simulink model "HysteresisFieldOrientedControl"  (R2020a)
settings: Solver=VariableStepAuto  StartTime=0.0  StopTime=10.0  RelTol=1e-3
libraries: simulink x1, powerlib_meascontrol x1
settings Model: Creator=Sony  LastModifiedBy=Sony

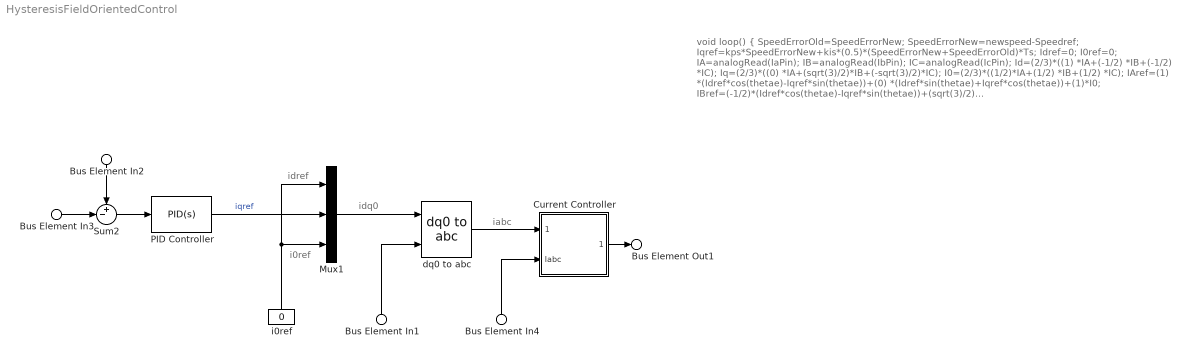
== system HysteresisFieldOrientedControl ==
  note: iabc
  note: idq0
  note: void loop()
      | {
      |   SpeedErrorOld=SpeedErrorNew;
      |   SpeedErrorNew=newspeed-Speedref;
      |
      |   Iqref=kps*SpeedErrorNew+kis*(0.5)*(SpeedErrorNew+SpeedErrorOld)*Ts;
      |   Idref=0;
      |   I0ref=0;
      |
      |   IA=analogRead(IaPin);
      |   IB=analogRead(IbPin);
      |   IC=analogRead(IcPin);
      |
      |   Id=(2/3)*((1)  *IA+(-1/2)     *IB+(-1/2)      *IC);
      |   Iq=(2/3)*((0)  *IA+(sqrt(3)/2)*IB+(-sqrt(3)/2)*IC);
      |   I0=(2/3)*((1/2)*IA+(1/2)      *IB+(1/2)       *IC);
      |
      |   IAref=(1)   *(Idref*cos(thetae)-Iqref*sin(thetae))+(0)         *(Idref*sin(thetae)+Iqref*cos(thetae))+(1)*I0;
      |   IBref=(-1/2)*(Idref*cos(thetae)-Iqref*sin(thetae))+(sqrt(3)/2) *(Idref*sin(thetae)+Iqref*cos(thetae))+(1)*I0;
      |   ICref=(-1/2)*(Idref*cos(thetae)-Iqref*sin(thetae))+(-sqrt(3)/2)*(Idref*sin(thetae)+Iqref*cos(thetae))+(1)*I0;
      |
      |   gatesignal=B000;
      |   if (IAref-IA>tolerance){gatesignal|=(1<<2);}
      |   if (-IAref+IA>tolerance){gatesignal|=(0<<2);}
      |   if (IBref-IB>tolerance){gatesignal|=(1<<1);}
      |   if (-IBref+IB>tolerance){gatesignal|=(0<<1);}
      |   if (ICref-IC>tolerance){gatesignal|=(1<<0);}
      |   if (-ICref+IC>tolerance){gatesignal|=(0<<0);}
      |   writeState(gatesignal);delayMicroseconds(Ts);
      | }
  note: i0ref
  note: idref
  Bus Element In1 : Inport  PortName=Rotor Electrical Angle
  Bus Element In4 : Inport  Port=2  PortName=Sampled Stator IABC
  Bus Element In3 : Inport  Port=3  PortName=Sampled Speed (rpm)
  Bus Element In2 : Inport  Port=4  PortName=Sampled Reference Speed (rpm)
  Current Controller : Subsystem
  Mux1 : Mux  Inputs=3
  PID Controller : simulink/Continuous/PID Controller  Controller=PID  Form=Parallel  TimeDomain=Continuous-time  UseExternalTs=off  SampleTime=1  IntegratorMethod=Forward Euler  FilterMethod=Forward Euler  ControllerParametersSource=internal  P=1  I=10  D=0  UseFilter=on  N=100  TunerSelectOption=Transfer Function Based (PID Tuner App)  InitialConditionSource=internal  InitialConditionForIntegrator=0  InitialConditionForFilter=0  DifferentiatorICPrevScaledInput=0  ExternalReset=none  TrackingMode=off  Kt=1  LimitOutput=on  UpperSaturationLimit=100  LowerSaturationLimit=-100  LinearizeAsGain=on  AntiWindupMode=clamping  Kb=1  POutMin=[]  POutMax=[]  IOutMin=[]  IOutMax=[]  DOutMin=[]  DOutMax=[]  NOutMin=[]  NOutMax=[]  SumOutMin=[]  SumOutMax=[]  SaturationOutMin=[]  SaturationOutMax=[]  PParamMin=[]  PParamMax=[]  IParamMin=[]  IParamMax=[]  DParamMin=[]  DParamMax=[]  NParamMin=[]  NParamMax=[]  KbParamMin=[]  KbParamMax=[]  KtParamMin=[]  KtParamMax=[]  KbOutMin=[]  KbOutMax=[]  KtOutMin=[]  KtOutMax=[]  IntegratorOutMin=[]  IntegratorOutMax=[]  FilterOutMin=[]  FilterOutMax=[]  SumI1OutMin=[]  SumI1OutMax=[]  SumI2OutMin=[]  SumI2OutMax=[]  SumI3OutMin=[]  SumI3OutMax=[]  SumI4OutMin=[]  SumI4OutMax=[]  SumDOutMin=[]  SumDOutMax=[]  DifferentiatorOutMin=[]  DifferentiatorOutMax=[]  FilterDiffOutCoefMin=[]  FilterDiffOutCoefMax=[]  ReciprocalOutMin=[]  ReciprocalOutMax=[]  SumDenOutMin=[]  SumDenOutMax=[]  SumNumOutMin=[]  SumNumOutMax=[]  DivideOutMin=[]  DivideOutMax=[]  UdiffTsProdOutMin=[]  UdiffTsProdOutMax=[]  NTsProdOutMin=[]  NTsProdOutMax=[]  UintegralTsProdOutMin=[]  UintegralTsProdOutMax=[]  UngainTsProdOutMin=[]  UngainTsProdOutMax=[]  IntegratorContinuousStateAttributes=''  IntegratorStateMustResolveToSignalObject=off  IntegratorRTWStateStorageClass=Auto  FilterContinuousStateAttributes=''  FilterStateMustResolveToSignalObject=off  FilterRTWStateStorageClass=Auto  ParallelPVariant=InternalParameters  IdealPVariant=Disabled  IVariant=InternalParameters  DVariant=InternalParameters  IntegratorVariant=Continuous  SatVariant=Enabled  AWVariant=ContClampingParallel  PCopyVariant=Disabled  TRVariant=Disabled  FdbkBlocksVariant=Forward  IdealPFdbkVariant=Disabled  SatFdbkVariant=Disabled  DerivativeFilterVariant=ContFilter  NVariant=InternalParameters  NCopyVariant=Disabled  FilterICVariant=InternalICsFilter  IntegratorICVariant=InternalICs  ExternalResetVariant=Disabled  TRSumVariant=Passthrough  SumFdbkVariant=Disabled  SumVariant=Sum_PID  TsampFilterVariant=InternalTs  TsampNgainVariant=Passthrough  TsampIntegralVariant=Passthrough
  Sum2 : Sum  Inputs=+-|
  dq0 to abc : powerlib_meascontrol/Transformations/dq0 to abc  Alignment=Aligned with phase A axis
  i0ref : Constant  Value=0
  Bus Element Out1 : Outport  PortName=Gatings
  wires:
  Current Controller/1(Pulses) -> Bus Element Out1/1
  PID Controller/1 -> Mux1/2  "iqref"
  Bus Element In4/1 -> Current Controller/2(Iabc)
  Bus Element In1/1 -> dq0 to abc/2
  Bus Element In3/1 -> Sum2/2
  Sum2/1 -> PID Controller/1
  Bus Element In2/1 -> Sum2/1
  dq0 to abc/1 -> Current Controller/1(Iabc_ref)
  Mux1/1 -> dq0 to abc/1
  i0ref/1 -> Mux1/1, Mux1/3

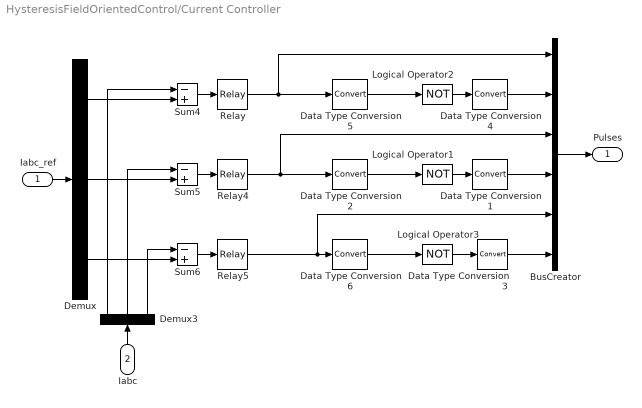
== system HysteresisFieldOrientedControl/Current Controller ==
  Iabc_ref : Inport
  Iabc : Inport  Port=2
  BusCreator : BusCreator  Inputs=6
  Data Type Conversion{1..6} (6 alike) : DataTypeConversion  SaturateOnIntegerOverflow=on  RndMeth=Zero
  Demux : Demux  Outputs=3
  Demux3 : Demux  Outputs=3
  Logical Operator1 : Logic  Operator=NOT
  Logical Operator2 : Logic  Operator=NOT
  Logical Operator3 : Logic  Operator=NOT
  Relay : Relay  OnSwitchValue=1/2  OffSwitchValue=-1/2
  Relay4 : Relay  OnSwitchValue=1/2  OffSwitchValue=-1/2
  Relay5 : Relay  OnSwitchValue=1/2  OffSwitchValue=-1/2
  Sum4 : Sum  Inputs=-+  InputSameDT=on  SaturateOnIntegerOverflow=on  OutDataTypeStr=Inherit: Same as first input
  Sum5 : Sum  Inputs=-+  InputSameDT=on  SaturateOnIntegerOverflow=on  OutDataTypeStr=Inherit: Same as first input
  Sum6 : Sum  Inputs=-+  InputSameDT=on  SaturateOnIntegerOverflow=on  OutDataTypeStr=Inherit: Same as first input
  Pulses : Outport
  wires:
  Iabc/1 -> Demux3/1
  Demux/2 -> Sum5/2
  Demux/1 -> Sum4/2
  Sum4/1 -> Relay/1
  Demux3/2 -> Sum5/1
  Demux3/1 -> Sum4/1
  Sum5/1 -> Relay4/1
  Demux3/3 -> Sum6/1
  Demux/3 -> Sum6/2
  Sum6/1 -> Relay5/1
  Iabc_ref/1 -> Demux/1
  Logical Operator2/1 -> Data Type Conversion4/1
  Data Type Conversion5/1 -> Logical Operator2/1
  Relay/1 -> BusCreator/1, Data Type Conversion5/1
  Data Type Conversion4/1 -> BusCreator/2
  Logical Operator1/1 -> Data Type Conversion1/1
  Data Type Conversion2/1 -> Logical Operator1/1
  Data Type Conversion1/1 -> BusCreator/4
  Logical Operator3/1 -> Data Type Conversion3/1
  Data Type Conversion6/1 -> Logical Operator3/1
  Data Type Conversion3/1 -> BusCreator/6
  Relay4/1 -> BusCreator/3, Data Type Conversion2/1
  Relay5/1 -> BusCreator/5, Data Type Conversion6/1
  BusCreator/1 -> Pulses/1
